simulink model "y7s"  (R2023b)
settings: Solver=FixedStepAuto  StartTime=0.0  StopTime=10.0  FixedStep=0.001  RelTol=1e-3
settings Model: Creator=asus  LastModifiedBy=asus

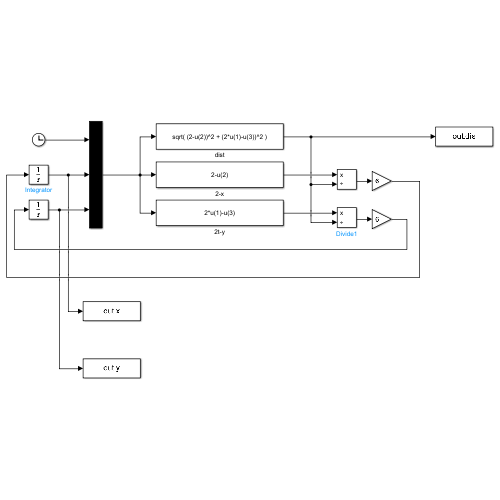
[thumbnail: Simulink's stored preview of the top-level diagram]
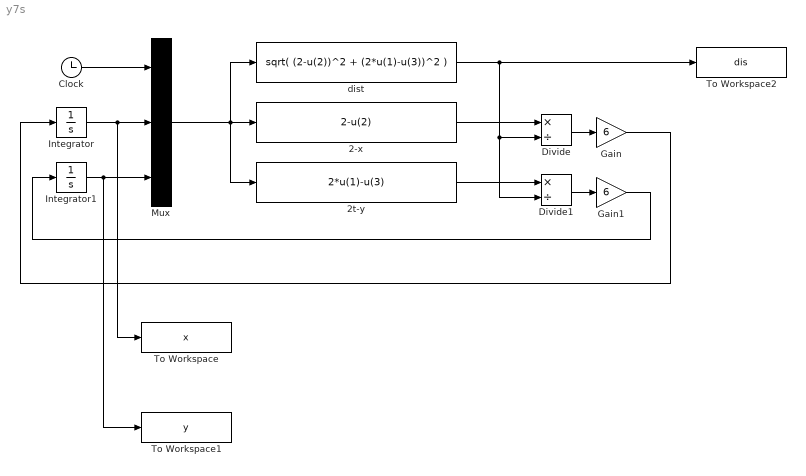
== system y7s ==
  2-x : Fcn  Expr=2-u(2)
  2t-y : Fcn  Expr=2*u(1)-u(3)
  Clock : Clock
  Divide : Product  Inputs=*/
  Divide1 : Product  Inputs=*/
  Gain : Gain  Gain=6
  Gain1 : Gain  Gain=6
  Integrator : Integrator
  Integrator1 : Integrator
  Mux : Mux  Inputs=3
  To Workspace : ToWorkspace  VariableName=x  SaveFormat=Timeseries  SampleTime=-1
  To Workspace1 : ToWorkspace  VariableName=y  SaveFormat=Timeseries  SampleTime=-1
  To Workspace2 : ToWorkspace  VariableName=dis  SaveFormat=Timeseries  SampleTime=-1
  dist : Fcn  Expr=sqrt( (2-u(2))^2 + (2*u(1)-u(3))^2 )
  wires:
  Integrator/1 -> To Workspace/1, Mux/2
  Clock/1 -> Mux/1
  Integrator1/1 -> To Workspace1/1, Mux/3
  Mux/1 -> 2t-y/1, 2-x/1, dist/1
  2-x/1 -> Divide/1
  dist/1 -> To Workspace2/1, Divide/2, Divide1/2
  2t-y/1 -> Divide1/1
  Divide/1 -> Gain/1
  Divide1/1 -> Gain1/1
  Gain/1 -> Integrator/1
  Gain1/1 -> Integrator1/1
